simulink model "chart_stateflow_2015"  (R2015a)
settings: Solver=ode45  StartTime=0.0  StopTime=10.0  RelTol=1e-3
settings Model: Creator=Administrator  LastModifiedBy=Administrator

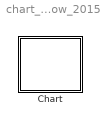
== system chart_stateflow_2015 ==
  Chart : Stateflow chart  TreatAsAtomicUnit=on

== stateflow chart chart_stateflow_2015/Chart ==
  state 报名阶段 [group]
  note: 
  state 校内审核
    state 学生报名
    学生报名 -> (junction 54) : 学生报名截止
    (junction 54) -> (junction 58) : 校内审核截止
  state 学校报名
  note: 1
  state 比赛阶段 [group]
    state 01
      note: 学校巡视
    state 02（grouped）
      note: 学生竞赛
      state 建模 [parallel]
        settings: executionOrder=1
      state 编程 [parallel]
        settings: executionOrder=2
      state 写论文 [parallel]
        settings: executionOrder=3
      state 吃饭 [parallel]
        settings: executionOrder=4
      state 睡觉 [parallel]
        settings: executionOrder=5
      state 上传 [parallel]
        settings: executionOrder=6
    (junction 67) -> 比赛阶段.01 [order 1]
    比赛阶段.01 -> (junction 80)
    02（grouped） -> (junction 80) : 竞赛结束
    (junction 67) -> 02（grouped） [order 2]
  note: 第一个人负责建模和编程
      | 第二个人负责写论文和上传论文
      | 我负责吃饭和睡觉
  state 分赛区评审阶段（grouped） [group]
    state 01
      note: 赛区一次评审送报
    state 02
      note: 全国评审
    state 03
      note: 赛区二次评审送报
    02 -> 03
    分赛区评审阶段（grouped）.01 -> 02
    (junction 71) -> 分赛区评审阶段（grouped）.01
    03 -> (junction 106) : 分赛区评审截止
  (junction 28) -> 学校报名 : 报名开始
  (junction 58) -> (junction 60) : 报名截止
  学校报名 -> 学生报名
  (junction 60) -> ?
  (default) -> (junction 67) [order 1] : 竞赛开赛
  (junction 80) -> ?
  (default) -> (junction 71) [order 2] : 评审开始
